simulink model "flightTestVehicle"  (Simulink 8.4)
settings: Solver=ode45  StartTime=0.0  StopTime=10.0  RelTol=1e-3
settings Model: Creator=brtaylor  LastModifiedBy=brtaylor
settings DataIOCC: SignalLoggingSaveFormat=Dataset
settings OptimizationCC: ExpressionDepthLimit=128
settings DebuggingCC: UnderspecifiedInitializationDetection=Simplified  MergeDetectMultiDrivingBlocksExec=error  FcnCallInpInsideContextMsg=EnableAllAsError  StateNameClashWarn=none
settings GRTTargetCC: CombineOutputUpdateFcns=on  GRTInterface=off

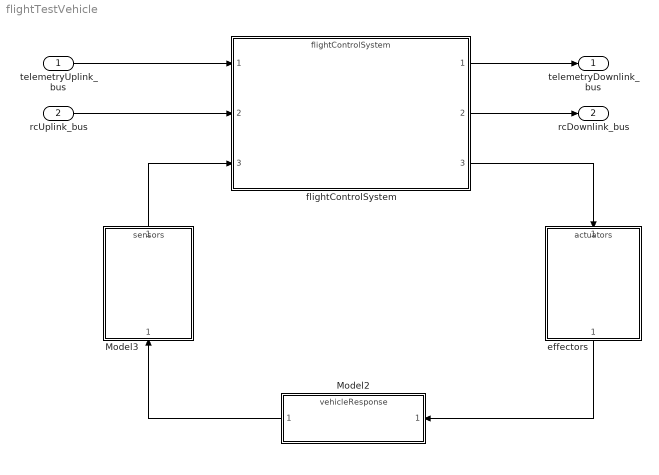
== system flightTestVehicle ==
  telemetryUplink_bus : Inport
  rcUplink_bus : Inport  Port=2
  Model2 : ModelReference  ModelNameDialog=vehicleResponse.mdl  SimulationMode=Normal  ModelReferenceVersion=1.1  CopyOfModelName=vehicleResponse.mdl  DefaultDataLogging=on
  Model3 : ModelReference  ModelNameDialog=sensors.mdl  SimulationMode=Normal  ModelReferenceVersion=1.1  CopyOfModelName=sensors.mdl  DefaultDataLogging=on
  effectors : ModelReference  ModelNameDialog=actuators.mdl  SimulationMode=Normal  ModelReferenceVersion=1.1  CopyOfModelName=actuators.mdl  DefaultDataLogging=on
      mask Display: image(imread('actuator.jpg'))
  flightControlSystem : ModelReference  ModelNameDialog=flightControlSystem.mdl  SimulationMode=Normal  ModelReferenceVersion=1.7  CopyOfModelName=flightControlSystem.mdl  DefaultDataLogging=on
      mask Display: image(imread('flightControlSystem.jpg'))
  telemetryDownlink_bus : Outport
  rcDownlink_bus : Outport  Port=2
  wires:
  telemetryUplink_bus/1 -> flightControlSystem/1
  rcUplink_bus/1 -> flightControlSystem/2
  flightControlSystem/1 -> telemetryDownlink_bus/1
  flightControlSystem/2 -> rcDownlink_bus/1
  flightControlSystem/3 -> effectors/1
  effectors/1 -> Model2/1
  Model3/1 -> flightControlSystem/3
  Model2/1 -> Model3/1
